simulink model "MATLABMobileReceiverExample"  (R2026a)
settings: Solver=VariableStepAuto  StopTime=inf
settings Model: Creator=dsportil  LastModifiedBy=dsportil
settings SimscapeCC: SimscapeNominalValues="[{\"value\":\"1\",\"unit\":\"A\"},{\"value\":\"1\",\"unit\":\"bar\"},{\"value\":\"1\",\"unit\":\"cm^2\"},{\"value\":\"1\",\"unit\":\"cm^3/s\"},{\"value\":\"1\",\"unit\":\"kJ/kg\"},{\"value\":\"1\",\"unit\":\"kW\"},{\"value\":\"1\",\"unit\":\"l\"},{\"value\":\"1\",\"unit\":\"N\"},{\"value\":\"1\",\"unit\":\"N*m\"},{\"value\":\"1\",\"unit\":\"V\"}]"  SimscapeLogType=none  SimscapeLogDataHistory=5000.0

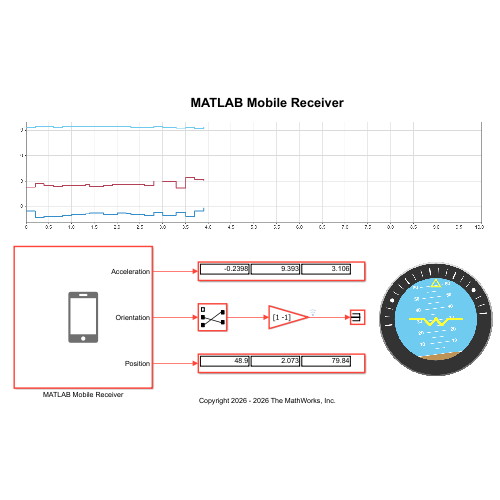
[thumbnail: Simulink's stored preview of the top-level diagram]
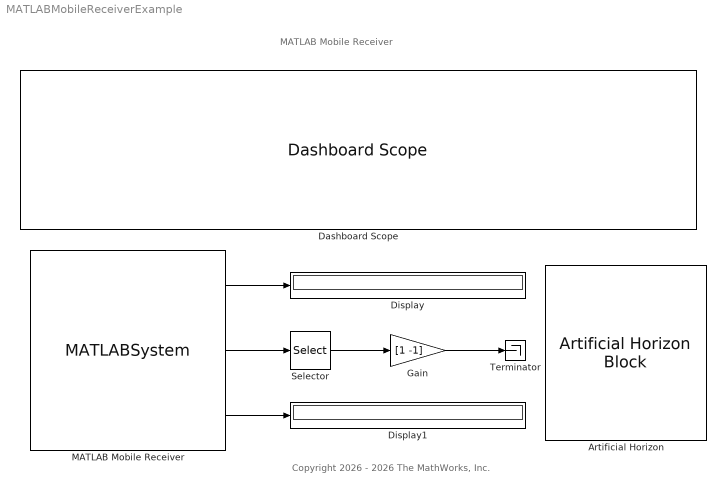
== system MATLABMobileReceiverExample ==
  note: Copyright 2026 - 2026 The MathWorks, Inc.
  note: MATLAB Mobile Receiver
  Artificial Horizon : ArtificialHorizonBlock  LabelPosition=Hide
  Dashboard Scope : DashboardScope  ShowInitialText=off  TimeSpan=10  Ymin=-10  Ymax=10  LegendPosition=Hide  UpdateMode=Scroll  FontColor=[0.0, 0.0, 0.0]
  Display : Display
  Display1 : Display
  Gain : Gain  Gain=[1 -1]
  MATLAB Mobile Receiver : MATLABSystem  System=classes.MATLABMobileReceiver  AccelerationEnabled=on  OrientationEnabled=on  AngularVelocityEnabled=off  PositionEnabled=on  MagneticFieldEnabled=off  Frequency=10  CameraEnabled=off  CameraSelected=back  FPS=1
      mask Type: classes.MATLABMobileReceiver
  Selector : Selector  InputPortWidth=3  IndexOptions=Index vector (dialog)  Indices=[3 2]  OutputSizes=1
  Terminator : Terminator
  wires:
  MATLAB Mobile Receiver/2 -> Selector/1
  MATLAB Mobile Receiver/1 -> Display/1
  Selector/1 -> Gain/1
  Gain/1 -> Terminator/1
  MATLAB Mobile Receiver/3 -> Display1/1
